simulink model "demo_kalman_msd"  (R2025a)
settings: Solver=VariableStepAuto  StartTime=0.0  StopTime=2  RelTol=1e-3
settings Model: Creator=xing2  LastModifiedBy=xing2

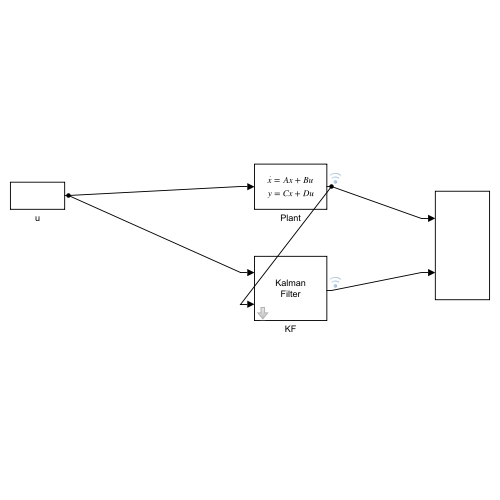
[thumbnail: Simulink's stored preview of the top-level diagram]
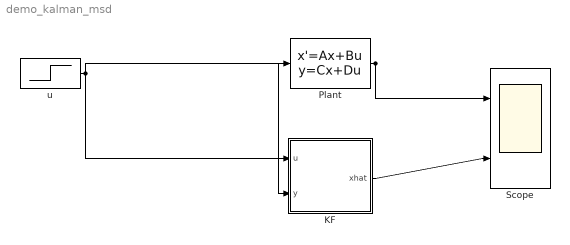
== system demo_kalman_msd ==
  KF : Subsystem  mask{A_kf=[0 1;-10 -0.5], B_aug=[0 3;1 5], C_kf=[1 0], D_aug=[0 0], x0=[0;0]}
      mask prompts: A_kf "A matrix"; B_aug "B_aug=[B K]"; C_kf "C matrix"; D_aug "D matrix"
      mask help: Kalman Filter. B_aug=[B, K_kalman] for input [u; y]
      mask Display: disp('Kalman\nFilter');
  Plant : StateSpace  A=[0 1;-10 -0.5]  B=[0;1]  C=[1 0]  D=0  InitialCondition=0
  Scope : Scope  NumInputPorts=2
  u : Step  Time=0.5  SampleTime=0
  wires:
  u/1 -> Plant/1, KF/1(u)
  Plant/1 -> KF/2(y), Scope/1
  KF/1(xhat) -> Scope/2

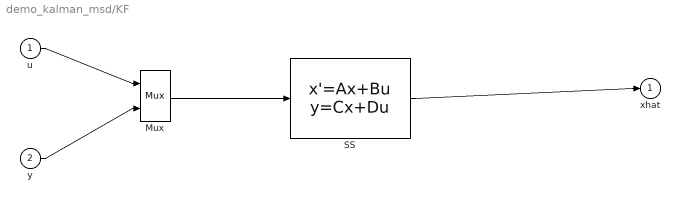
== system demo_kalman_msd/KF ==
  u : Inport
  y : Inport  Port=2
  Mux : Mux  Inputs=2
  SS : StateSpace  A=A_kf  B=B_aug  C=C_kf  D=D_aug  InitialCondition=x0
  xhat : Outport
  wires:
  SS/1 -> xhat/1
  Mux/1 -> SS/1
  y/1 -> Mux/2
  u/1 -> Mux/1
